simulink model "THREE_PHASE_INVERTER_AND_VFD"  (R2018b)
settings: Solver=VariableStepAuto  StartTime=0.0  StopTime=10.0  RelTol=1e-3
libraries: powerlib x10, simulink x3, powerlib_meascontrol x1
settings Model: Creator=dmait  LastModifiedBy=dmait

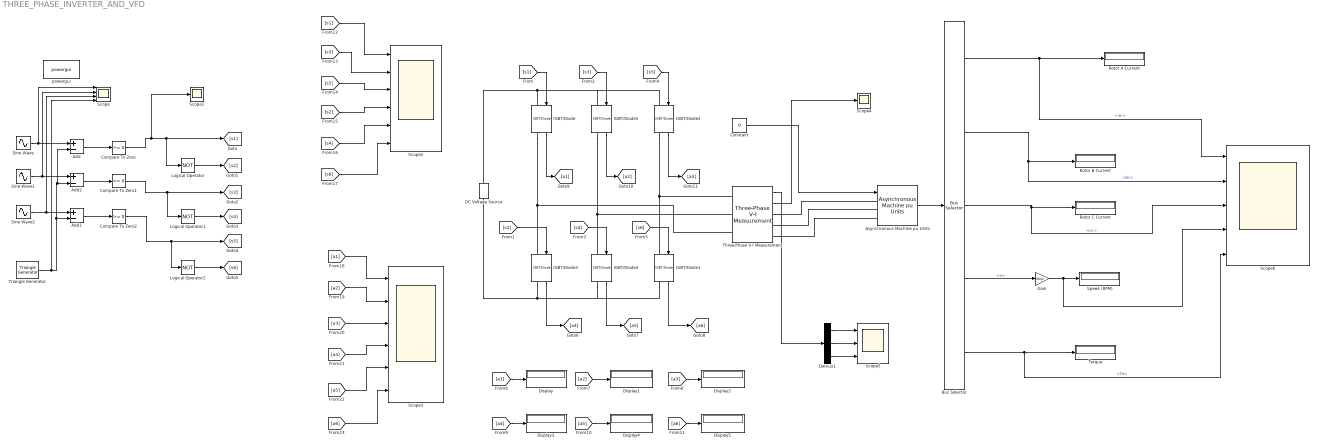
== system THREE_PHASE_INVERTER_AND_VFD ==
  Add : Sum  Inputs=+-
  Add1 : Sum  Inputs=+-
  Add2 : Sum  Inputs=+-
  Asynchronous Machine pu Units : powerlib/Machines/Asynchronous Machine pu Units  RotorType=Squirrel-cage  PresetModel="01:  5 HP   460 V 60Hz 1750 RPM"  MechanicalLoad=Torque Tm  ShowDetailedParameters=on  ReferenceFrame=Rotor  Units=pu  MeasurementBus=on  NominalParameters=[3730 460 60]  Stator=[0.01965 0.0397]  Rotor=[0.01909 0.0397]  Cage1=[0.01909 0.0397]  Cage2=[0.01909 0.0397]  Lm=1.354  Mechanical=[0.09526 0.05479 2]  PolePairs=2  InitialConditions="[ 1,0   0,0,0   0,0,0 ]"  SimulateSaturation=off  Saturation="[0.212,0.4201,0.8125,1.0979,1.4799,2.2457,3.2586,4.5763,6.4763 ;   0.5,0.7,0.9,1,1.1,1.2 ,1.3,1.4,1.5]"  LoadFlowParameters=0  TsPowergui=0  TsBlock=-1  IterativeModel=Trapezoidal non iterative  IterativeDiscreteModel=Trapezoidal non iterative  Pmec=0
      settings: SourceProductName=Simscape Power Systems  SourceProductBaseCode=PS
  Bus Selector : BusSelector  OutputSignals=iar,ibr,icr,w,Te
  Compare To Zero : simulink/Logic and Bit Operations/Compare To Zero  relop=>=  OutDataTypeStr=boolean
  Compare To Zero1 : simulink/Logic and Bit Operations/Compare To Zero  relop=>=  OutDataTypeStr=boolean
  Compare To Zero2 : simulink/Logic and Bit Operations/Compare To Zero  relop=>=  OutDataTypeStr=boolean
  Constant : Constant  Value=0
  DC Voltage Source : powerlib/Electrical Sources/DC Voltage Source  Amplitude=500  Measurements=None
  Demux1 : Demux  Outputs=3
  Display{,1..5} (6 alike) : Display
  Gain : Gain  Gain=30/pi
  IGBT/Diode{,1..5} (6 alike) : powerlib/Power Electronics/IGBT//Diode  Ron=1e-3  Rs=1e5  Cs=inf  Measurements=on
  Logical Operator : Logic  Operator=NOT  AllPortsSameDT=off  OutDataTypeStr=boolean
  Logical Operator1 : Logic  Operator=NOT  AllPortsSameDT=off  OutDataTypeStr=boolean
  Logical Operator2 : Logic  Operator=NOT  AllPortsSameDT=off  OutDataTypeStr=boolean
  Rotor A Current : Display
  Rotor B Current : Display
  Rotor C Current : Display
  Scope : Scope  NumInputPorts=4
  Scope1 : Scope
  Scope2 : Scope  NumInputPorts=6
  Scope3 : Scope  NumInputPorts=6
  Scope4 : Scope
  Scope5 : Scope  NumInputPorts=3
  Scope6 : Scope  NumInputPorts=5
  Sine Wave : Sin  Frequency=2*pi*50  SampleTime=0
  Sine Wave1 : Sin  Frequency=2*pi*50  Phase=2*pi/3  SampleTime=0
  Sine Wave2 : Sin  Frequency=2*pi*50  Phase=4*pi/3  SampleTime=0
  Speed (RPM) : Display
  Three-Phase V-I Measurement : powerlib/Measurements/Three-Phase V-I Measurement  VoltageMeasurement=phase-to-phase  SetLabelV=off  LabelV=Vabc  Vpu=off  VpuLL=off  CurrentMeasurement=yes  SetLabelI=off  LabelI=Iabc  Ipu=off  Pbase=100e6  Vbase=500e3  OutputType=Complex  PhasorSimulation=off  PSBequivalent=0
  Torque : Display
  Triangle Generator : powerlib_meascontrol/Pulse & Signal Generators/Triangle Generator  Freq=500  Phase=180  Ts=0
  powergui : powerlib/powergui  Priority=1  SimulationMode=Continuous  SampleTime=50e-6  frequency=60  Iterations=50  frequencyindice=0  Pbase=100e6  ErrMax=1e-4  UnitsV=kV  UnitsW=MW  buscounter=0  FunctionMessages=off  echomessages=off  EnableUseOfTLC=off  CurrentSourceSwitches=off  DisableSnubberDevices=off  DisableRonSwitches=off  DisableVfSwitches=off  DisplayEquations=off  SolverType=Tustin/Backward Euler (TBE)  Interpol=off  ExternalGateDelay=off  methode=off  Ts=100  x0status=blocks  SPID=on  SwTol=0  HookPort=off  RestoreLinks=warning  ResistiveCurrentMeasurement=off  Frange=[0:2:500]  Ylog=off  Xlog=on  ShowGrid=off  save=off  variable=ZData  structure=0  ZoomFFT=off  StartTime=0.0  cycles=1  DisplayStyle=1  fundamental=60  FreqAxis=off  MaxFrequency=1000  frequencyindicesteady=1  RmsSteady=1  display=off
  wires:
  Sine Wave/1 -> Add/1, Scope/1
  Sine Wave1/1 -> Add2/1, Scope/2
  Sine Wave2/1 -> Add1/1, Scope/3
  Triangle Generator/1 -> Scope/4, Add/2, Add2/2, Add1/2
  Add/1 -> Compare To Zero/1
  Add2/1 -> Compare To Zero1/1
  Add1/1 -> Compare To Zero2/1
  Compare To Zero/1 -> Scope1/1, Logical Operator/1, [s1]
  Logical Operator/1 -> [s2]
  Compare To Zero1/1 -> Logical Operator1/1, [s3]
  Logical Operator1/1 -> [s4]
  Compare To Zero2/1 -> Logical Operator2/1, [s5]
  Logical Operator2/1 -> [s6]
  [s1] -> IGBT/Diode/1
  [s3] -> IGBT/Diode5/1
  [s5] -> IGBT/Diode2/1
  [s2] -> IGBT/Diode3/1
  [s4] -> IGBT/Diode4/1
  [s6] -> IGBT/Diode1/1
  [a1] -> Display/1
  [a5] -> Display4/1
  [a4] -> Display3/1
  [a3] -> Display2/1
  [a2] -> Display1/1
  [a6] -> Display5/1
  IGBT/Diode/1 -> [a1]
  IGBT/Diode5/1 -> [a2]
  IGBT/Diode2/1 -> [a3]
  IGBT/Diode3/1 -> [a4]
  IGBT/Diode4/1 -> [a5]
  IGBT/Diode1/1 -> [a6]
  [s1] -> Scope2/1
  [s3] -> Scope2/2
  [s5] -> Scope2/3
  [s2] -> Scope2/4
  [s4] -> Scope2/5
  [s6] -> Scope2/6
  [a1] -> Scope3/1
  [a2] -> Scope3/2
  [a3] -> Scope3/3
  [a4] -> Scope3/4
  [a5] -> Scope3/5
  [a6] -> Scope3/6
  Constant/1 -> Asynchronous Machine pu Units/1
  Three-Phase V-I Measurement/2 -> Scope4/1
  Demux1/1 -> Scope5/1
  Three-Phase V-I Measurement/1 -> Demux1/1
  Demux1/2 -> Scope5/2
  Demux1/3 -> Scope5/3
  Bus Selector/2 -> Rotor B Current/1, Scope6/2  "<ibr>"
  Bus Selector/3 -> Rotor C Current/1, Scope6/3  "<icr>"
  Bus Selector/5 -> Torque/1, Scope6/5  "<Te>"
  Gain/1 -> Scope6/4, Speed (RPM)/1
  Asynchronous Machine pu Units/1 -> Bus Selector/1
  Bus Selector/1 -> Scope6/1, Rotor A Current/1  "<iar>"
  Bus Selector/4 -> Gain/1  "<w>"
  connections:
  IGBT/Diode/RConn1 -- IGBT/Diode3/LConn1 -- Three-Phase V-I Measurement/LConn3
  IGBT/Diode5/RConn1 -- Three-Phase V-I Measurement/LConn2 -- IGBT/Diode4/LConn1
  IGBT/Diode2/RConn1 -- Three-Phase V-I Measurement/LConn1 -- IGBT/Diode1/LConn1
  DC Voltage Source/RConn1 -- IGBT/Diode2/LConn1 -- IGBT/Diode5/LConn1 -- IGBT/Diode/LConn1
  DC Voltage Source/LConn1 -- IGBT/Diode1/RConn1 -- IGBT/Diode4/RConn1 -- IGBT/Diode3/RConn1
  Three-Phase V-I Measurement/RConn1 -- Asynchronous Machine pu Units/LConn1
  Three-Phase V-I Measurement/RConn2 -- Asynchronous Machine pu Units/LConn2
  Three-Phase V-I Measurement/RConn3 -- Asynchronous Machine pu Units/LConn3
